simulink model "PV_MEV"  (R2025a)
settings: Solver=VariableStepAuto  StartTime=0.0  StopTime=1  RelTol=1e-3
InitFcn:
  | init_paras
model workspace (MAT data in the model file):
  atk_params = [0 1 0.85 999 0 50 0 0]
  atk_params_vdc = [0 1 0.85 999 0 50 0 0]
values from neighbouring files (symbols this model uses):
  C_PFC = 2600e-6    (= 0.0026)    [init_paras.m]
  ENABLE_HIL = 0    [init_paras.m]
  estimation_src = 1    [init_paras.m]
  Fnom = 50    [init_paras.m]
  Fr_I = Fnom*2    (= 100)    [init_paras.m]
  Ki_V = 80    [init_paras.m]
  Kp_I = 0.06    [init_paras.m]
  Kp_V = 0.25    [init_paras.m]
  Kr_I = 2.5    [init_paras.m]
  L_PFC = 600e-6    (= 0.0006)    [init_paras.m]
  Limit_V = 100    [init_paras.m]
  mm_10cycle_points = mm_points_per_cycle * 10    (= 800)    [init_paras.m]
  mm_fund_freq = 50    [init_paras.m]
  mm_points_per_cycle = 80    [init_paras.m]
  RL_PFC = 20e-3    (= 0.02)    [init_paras.m]
  Ro = 22.22    [init_paras.m]
  Ts_Control = 1/Fc    (= 5e-05)    [init_paras.m]
  Ts_Power = 50e-9    (= 5e-08)    [init_paras.m]
  use_d_predict = 1    [init_paras.m]
  use_harmonic = 1    [init_paras.m]
  use_p_predict = 0    [init_paras.m]
  Vnom_ac = 240    [init_paras.m]
undefined symbols (not defined in the file or in its folder): D1, Delta, DiscIntNeverNeededParam
libraries: spsSeriesRLCBranchLib x17, spsMeanLib x16, spsCurrentMeasurementLib x9, spsFourierLib x8, spsTHDLib x8, spsVoltageMeasurementLib x8, spsDiodeLib x7, MyLibrary x6, instrumentlib x6, pycoexlib x6, simulink x6, spsPWMGeneratorDCDCLib x4
(part 4 of 6)

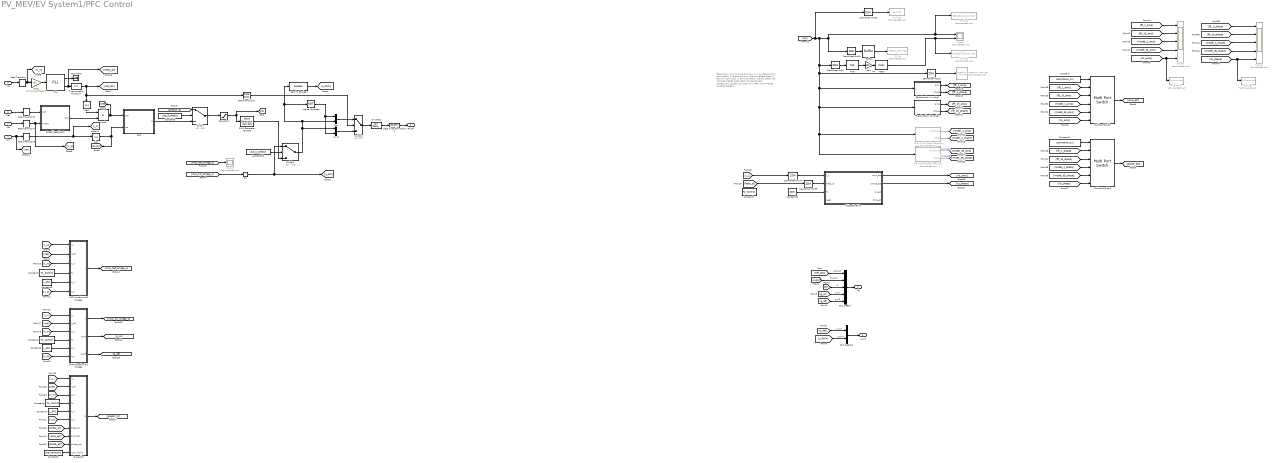
== system PV_MEV/EV System1/PFC Control ==
  note: Make sure
      | 1. onnxruntime and onnx in your base python enviroment.
      | 2. reload the onnx file and refresh them in the onnx call block.
      | or comment them like this
      | otherwise will lead matlab crash
      |
      | (bash)
      | conda activate matlab_onnx_py310
      | pip install onnx==1.14.0
      |
      | (matlab console)
      | target = "/home/changhong/anaconda3/envs/matlab_onnx_py310/bin/python";
      | pe = pyenv
      | pyenv("Version", target)
  Vref : Inport
  Vdc : Inport  Port=2
  Vac : Inport  Port=3
  Iac : Inport  Port=4
  AbsI : Abs  SaturateOnIntegerOverflow=off
  AbsV : Abs  SaturateOnIntegerOverflow=off
  Buffer : Buffer  N=80  V=79  OutputFrames=off
  Bus Creator : BusCreator  Inputs=5
  Bus Creator1 : BusCreator  Inputs=2
  Cast To Boolean : DataTypeConversion  OutDataTypeStr=boolean  SaturateOnIntegerOverflow=off  RndMeth=Floor
  Constant : Constant  Value=estimation_src
  Constant{1..2,4,6} (4 alike) : Constant  Value=Ts_Control
  Constant10 : Constant  Value=use_p_predict
  Constant11 : Constant  Value=estimation_src
  Constant12 : Constant  Value=4000
  Constant3 : Constant  Value=L_PFC
  Constant5 : Constant  Value=L_PFC
  Constant7 : Constant  Value=L_PFC
  Constant8 : Constant  Value=use_harmonic
  Constant9 : Constant  Value=use_d_predict
  D_predict : MATLAB Function  TreatAsAtomicUnit=on
  Data Type Conversion2 : DataTypeConversion  OutDataTypeStr=double  SaturateOnIntegerOverflow=off  RndMeth=Floor
  Gain : Gain  Gain=100
  Half Cycle Model Prediction : Subsystem  Commented=on
  Logical Operator : Logic  Operator=NOT  AllPortsSameDT=off  OutDataTypeStr=float('double')
  MCP Function Half bridge1 : MATLAB Function  TreatAsAtomicUnit=on
  Mean : spsMeanLib/Mean  Freq=50  Vinit=0  Ts=1/4000
  Multiport Switch : MultiPortSwitch  Inputs=5  SaturateOnIntegerOverflow=off  InputSameDT=off
  Multiport Switch1 : MultiPortSwitch  Inputs=5  SaturateOnIntegerOverflow=off  InputSameDT=off
  Mux : Mux  Inputs=2
  Mux2 : Mux  Inputs=2
  On Delay : spsOnDelayLib/On Delay  DelayType=On delay  delay=DT_PFC  ic=0  Ts=Ts_Power
  One  Cycle Model Prediction : Subsystem  Commented=on
  PLL : spsPLLLib/PLL  Fmin=0.9*Fnom  Par_Init=[0, Fnom]  ParK=[180, 3200, 1]  TcD=1e-4  MaxRateChangeFreq=12  FilterCutOffFreq=25  Ts=Ts_Control  AGC=on
  PR2 : Subsystem  mask(Current Regulator (Pr)){Kp=Kp_I, Kr=Kr_I, Fr=Fr_I}
      mask prompts: Kp "Proportional gain"; Kr "Resonant gain"; Fr "Resonant frequency (Hz)"
      mask help: This block implements a currentregulator using a PR controller.
      mask Display: disp('Current Regulator\n PR');
  PWM Generator (DC-DC) : spsPWMGeneratorDCDCLib/PWM Generator (DC-DC)  Fsw=Fsw  Ts=Ts_Power
  Prod1 : Product
  RLS_estimation : MATLAB Function  TreatAsAtomicUnit=on
  RT : RateTransition  OutPortSampleTime=5e-08
  Rate Transition{,3..5} (4 alike) : RateTransition  OutPortSampleTime=Ts_Control
  Rate Transition2 : RateTransition  OutPortSampleTime=Ts_Power
  Saturation : Saturate  UpperLimit=1  LowerLimit=0
  Scope : Scope  Commented=on  NumInputPorts=2
      settings: ActiveDisplayYMinimum=-211.219  ActiveDisplayYMaximum=223.7073  DataLoggingVariableName=ScopeData4  DataLoggingSaveFormat=Array
  Scope1 : Scope  Commented=on  NumInputPorts=5
      settings: ActiveDisplayYMinimum=-19.4864  ActiveDisplayYMaximum=175.3777  DataLoggingVariableName=ScopeData5  DataLoggingSaveFormat=Array
  Scope2 : Scope  Commented=on
      settings: DataLoggingVariableName=ScopeData9  DataLoggingSaveFormat=Array
  Scope3 : Scope  Commented=on  NumInputPorts=5
      settings: ActiveDisplayYMinimum=-3.927  ActiveDisplayYMaximum=3.927  DataLoggingVariableName=ScopeData6  DataLoggingSaveFormat=Array
  Spectrum Analyzer : SpectrumAnalyzer  Commented=on  WindowPosition=[-2559.000000,62.000000,1707.000000,996.000000,]  ScopeFrameLocation=window  SampleRateSource=Property  SampleRate=8000  PlotAsTwoSidedSpectrum=off  WindowInvariantSamplesPerUpdate=on  FrequencySpan=Start and stop frequencies  StartFrequency=0  StopFrequency=2000  YLimits=[-21.57310057,75.63654601]  ColorLimits=[-42.4528 59.157]
  Speed Regulator2 : Subsystem  DialogController=POWERSYS.PowerSysDialog  mask(Voltage Regulator){Kp=Kp_V, Ki=Ki_V, Limit_wreg=Limit_V, Init=0, Ts=Ts_Control}
      mask prompts: Kp "Proportional gain (Kp):"; Ki "Integral gain (Ki):"; Limit_wreg "Output limits"; Init "Output initial value:"; Ts "Sample time:"
      mask help: This block implements a voltage regulator using an ant-windup PI controller.
      mask Display: disp('Voltage\nRegulator');
  Switch : Switch  Criteria=u2 > Threshold  Threshold=0.5  SaturateOnIntegerOverflow=off  InputSameDT=off
  Switch1 : Switch  SaturateOnIntegerOverflow=off  InputSameDT=off
  Switch2 : Switch  Criteria=u2 > Threshold  Threshold=0.5  SaturateOnIntegerOverflow=off  InputSameDT=off
  THD : spsTHDLib/THD  Freq=50  Ts=1/4000
  Terminator : Terminator
  To File : ToFile  Commented=on  Filename=MPCC_IAC.mat  SaveFormat=Timeseries
  To File1 : ToFile  Commented=on  Filename=rls_phase.mat  SaveFormat=Timeseries
  To File2 : ToFile  Commented=on  Filename=rls_amp.mat  SaveFormat=Timeseries
  To File3 : ToFile  Commented=on  Filename=Iac.mat  SaveFormat=Timeseries
  To File4 : ToFile  Commented=on  Filename=results/Iac_ori.mat  SaveFormat=Timeseries
  To File5 : ToFile  Commented=on  Filename=results/THD_ori.mat  SaveFormat=Timeseries
  Trigonometric Function7 : Trigonometry
  UMPC Function Full bridge1 : MATLAB Function  TreatAsAtomicUnit=on
  Zero-Order Hold{,1,3..5} (5 alike) : ZeroOrderHold  SampleTime=1/4000
  Zero-Order Hold2 : ZeroOrderHold  SampleTime=1/8000
  fft estimation 1 cycle2 : Subsystem
  fft estimation 10 cycle2 : Subsystem
  to-pu : Gain  Gain=1/(Vnom_ac*sqrt(2))
  g1_g2 : Outport  PortDimensions=2
  Sig : Outport  Port=2
  u_swt : Outport  Port=3
  wires:
  Zero-Order Hold5/1 -> RLS_estimation/2(theta_pll)
  Zero-Order Hold4/1 -> RLS_estimation/1(i_L)
  Constant12/1 -> RLS_estimation/3(Ts)
  [i_L] -> Zero-Order Hold4/1
  Zero-Order Hold3/1 -> To File3/1
  [rls_phase] -> Scope3/5, To File1/1
  [model_05_phase] -> Scope3/4
  [model_1_phase] -> Scope3/3
  [fft_10_phase] -> Scope3/2
  [fft_1_phase] -> Scope3/1
  [rls_amp] -> Scope1/5, To File2/1
  [model_05_amp] -> Scope1/4
  [model_1_amp] -> Scope1/3
  [fft_10_amp] -> Scope1/2
  [fft_1_amp] -> Scope1/1
  Constant11/1 -> Multiport Switch1/1
  Multiport Switch1/1 -> [phase_est]
  [fft_1_phase] -> Multiport Switch1/2
  [fft_10_phase] -> Multiport Switch1/3
  [model_1_phase] -> Multiport Switch1/4
  [model_05_phase] -> Multiport Switch1/5
  [rls_phase] -> Multiport Switch1/6
  [rls_amp] -> Multiport Switch/6
  [model_05_amp] -> Multiport Switch/5
  [model_1_amp] -> Multiport Switch/4
  [fft_10_amp] -> Multiport Switch/3
  [fft_1_amp] -> Multiport Switch/2
  RLS_estimation/2(phase_est) -> [rls_phase]
  RLS_estimation/1(amp_est) -> [rls_amp]
  Multiport Switch/1 -> [amp_est]
  Half Cycle Model Prediction/2(phase) -> [model_05_phase]  "hase_est"
  Half Cycle Model Prediction/1(amplitude) -> [model_05_amp]  "amp_est"
  One  Cycle Model Prediction/2(phase) -> [model_1_phase]
  One  Cycle Model Prediction/1(amplitude) -> [model_1_amp]
  fft estimation 10 cycle2/2(phase) -> [fft_10_phase]
  fft estimation 10 cycle2/1(amp) -> [fft_10_amp]
  fft estimation 1 cycle2/2(phase) -> [fft_1_phase]
  fft estimation 1 cycle2/1(amp) -> [fft_1_amp]
  Constant/1 -> Multiport Switch/1
  Logical Operator/1 -> Mux/1, Mux2/2
  Constant10/1 -> Switch2/2
  Switch/1 -> Saturation/1
  PR2/1(D) -> Switch/3
  [predict_D] -> Switch/1
  Constant9/1 -> Switch/2
  [mcp_half_bridge_o] -> Scope2/1
  D_predict/1(D) -> [predict_D]
  [theta_pll] -> D_predict/7(theta_pll)
  Constant8/1 -> D_predict/10(use_harmonic)
  [phase_est] -> D_predict/9(phase_est)
  [amp_est] -> D_predict/8(amp_est)
  [V_o] -> D_predict/6(V_o)
  Constant7/1 -> D_predict/5(L_in)
  Constant6/1 -> D_predict/4(Ts)
  [V_in] -> D_predict/3(V_in)
  [Iref] -> D_predict/2(i_ref)
  [i_L] -> D_predict/1(i_L)
  [theta_pll] -> Zero-Order Hold5/1
  [g_off] -> Bus Creator/5  "g_off"
  [g_on] -> Bus Creator/4  "g_on"
  UMPC Function Full bridge1/3(g_off) -> [g_off]
  UMPC Function Full bridge1/2(g_on) -> [g_on]
  UMPC Function Full bridge1/1(y) -> [mcp_full_bridge_o]
  [V_o] -> UMPC Function Full bridge1/6(V_o)
  Constant5/1 -> UMPC Function Full bridge1/5(L_in)
  Constant4/1 -> UMPC Function Full bridge1/4(Ts)
  [V_in] -> UMPC Function Full bridge1/3(V_in)
  [Iref] -> UMPC Function Full bridge1/2(i_ref)
  [i_L] -> UMPC Function Full bridge1/1(i_L)
  MCP Function Half bridge1/1(y) -> [mcp_half_bridge_o]
  [V_o] -> MCP Function Half bridge1/6(V_o)
  Constant3/1 -> MCP Function Half bridge1/5(L_in)
  Constant2/1 -> MCP Function Half bridge1/4(Ts)
  [V_in] -> MCP Function Half bridge1/3(V_in)
  [Iref] -> MCP Function Half bridge1/2(i_ref)
  [i_L] -> MCP Function Half bridge1/1(i_L)
  Zero-Order Hold1/1 -> Buffer/1
  THD/1 -> Gain/1
  Zero-Order Hold2/1 -> Spectrum Analyzer/1
  Mean/1 -> Scope/2, To File5/1
  Zero-Order Hold/1 -> THD/1
  Gain/1 -> Mean/1
  Buffer/1 -> To File/1
  [Iac] -> Scope/1, To File4/1, Zero-Order Hold1/1, Zero-Order Hold/1, Zero-Order Hold2/1, fft estimation 1 cycle2/1(u), fft estimation 10 cycle2/1(u), One  Cycle Model Prediction/1(u), Half Cycle Model Prediction/1(u), Zero-Order Hold3/1  "Iac"
  [u_PWM] -> Bus Creator1/2  "u_PWM"
  On Delay/1 -> Data Type Conversion2/1
  Vref/1 -> Rate Transition3/1
  Switch2/1 -> Mux2/1, Mux/2, Cast To Boolean/1, Logical Operator/1
  [Iac_abs] -> Bus Creator/2  "Iac_abc"
  AbsV/1 -> Prod1/1
  PLL/1 -> Terminator/1
  Rate Transition5/1 -> AbsI/1, [i_L]
  Bus Creator/1 -> Sig/1
  Prod1/1 -> PR2/1(Iref), [Iref]
  Vac/1 -> Rate Transition/1
  PWM Generator (DC-DC)/1 -> Switch2/3
  Cast To Boolean/1 -> [u_PWM]
  RT/1 -> [u_obs], Switch2/1
  [Iref_obs] -> Bus Creator/1  "Iref_obs"
  [mcp_full_bridge_o] -> RT/1
  Vdc/1 -> Rate Transition4/1
  Mux2/1 -> Switch1/3
  [u_obs] -> Bus Creator1/1  "u_obs"
  Rate Transition4/1 -> [V_o], Speed Regulator2/2(Vmeas)
  Switch1/1 -> On Delay/1
  Rate Transition3/1 -> Speed Regulator2/1(Vref)
  [D] -> Bus Creator/3  "D"
  Trigonometric Function7/1 -> [Iref_obs], Rate Transition2/1, AbsV/1
  AbsI/1 -> [Iac_abs], PR2/2(Iac)
  Bus Creator1/1 -> u_swt/1
  Rate Transition/1 -> to-pu/1, [V_in]
  to-pu/1 -> PLL/1
  Saturation/1 -> [D], PWM Generator (DC-DC)/1
  PLL/2 -> Trigonometric Function7/1, [theta_pll]
  Data Type Conversion2/1 -> g1_g2/1
  Rate Transition2/1 -> Switch1/2
  Speed Regulator2/1(Out) -> Prod1/2
  Iac/1 -> Rate Transition5/1, [Iac]
  Mux/1 -> Switch1/1

== system PV_MEV/EV System1/Subsystem ==

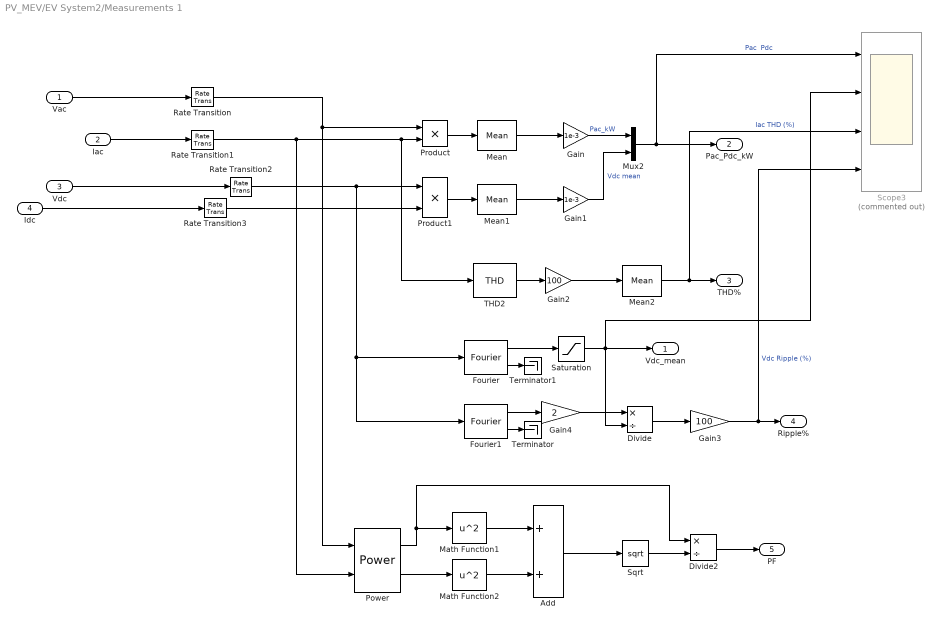
== system PV_MEV/EV System2/Measurements 1 ==
  Vac : Inport
  Iac : Inport  Port=2
  Vdc : Inport  Port=3
  Idc : Inport  Port=4
  Add : Sum
  Divide : Product  Inputs=*/
  Divide2 : Product  Inputs=*/
  Fourier : spsFourierLib/Fourier  Freq=Fnom  n=0  InInit=[0, 0]  Ts=Ts_Control
  Fourier1 : spsFourierLib/Fourier  Freq=Fnom  n=2  InInit=[0, 0]  Ts=Ts_Control
  Gain : Gain  Gain=1e-3
  Gain1 : Gain  Gain=1e-3
  Gain2 : Gain  Gain=100
  Gain3 : Gain  Gain=100
  Gain4 : Gain  Gain=2
  Math Function1 : Math  Operator=square
  Math Function2 : Math  Operator=square
  Mean : spsMeanLib/Mean  Freq=Fnom  Vinit=0  Ts=Ts_Control
  Mean1 : spsMeanLib/Mean  Freq=Fnom  Vinit=0  Ts=Ts_Control
  Mean2 : spsMeanLib/Mean  Freq=Fnom  Vinit=0  Ts=Ts_Control
  Mux2 : Mux  Inputs=2
  Power : spsPowerLib/Power  Freq=Fnom  Vinit=[1, 0]  Iinit=[1, 0]  Ts=Ts_Control
  Product : Product
  Product1 : Product
  Rate Transition{,1..3} (4 alike) : RateTransition  OutPortSampleTime=Ts_Control
  Saturation : Saturate  UpperLimit=inf  LowerLimit=eps
  Scope3 : Scope  Commented=on  NumInputPorts=4
      settings: DataLoggingSaveFormat=Array
  Sqrt : Sqrt
  THD2 : spsTHDLib/THD  Freq=Fnom  Ts=Ts_Control
  Terminator : Terminator
  Terminator1 : Terminator
  Vdc_mean : Outport
  Pac_Pdc_kW : Outport  Port=2
  THD% : Outport  Port=3
  Ripple% : Outport  Port=4
  PF : Outport  Port=5
  wires:
  Gain1/1 -> Mux2/2  "Vdc mean"
  Product1/1 -> Mean1/1
  Mean/1 -> Gain/1
  Product/1 -> Mean/1
  Gain/1 -> Mux2/1  "Pac_kW"
  THD2/1 -> Gain2/1
  Mean1/1 -> Gain1/1
  Iac/1 -> Rate Transition1/1
  Mux2/1 -> Scope3/1, Pac_Pdc_kW/1  "Pac  Pdc"
  Gain2/1 -> Mean2/1
  Mean2/1 -> Scope3/3, THD%/1  "Iac THD (%)"
  Fourier/2 -> Terminator1/1
  Fourier/1 -> Saturation/1
  Saturation/1 -> Scope3/2, Vdc_mean/1, Divide/2
  Divide/1 -> Gain3/1
  Fourier1/1 -> Gain4/1
  Gain4/1 -> Divide/1
  Fourier1/2 -> Terminator/1
  Gain3/1 -> Scope3/4, Ripple%/1  "Vdc Ripple (%)"
  Power/1 -> Math Function1/1, Divide2/1
  Power/2 -> Math Function2/1
  Math Function1/1 -> Add/1
  Math Function2/1 -> Add/2
  Add/1 -> Sqrt/1
  Sqrt/1 -> Divide2/2
  Divide2/1 -> PF/1
  Rate Transition1/1 -> Power/2, THD2/1, Product/2
  Vdc/1 -> Rate Transition2/1
  Idc/1 -> Rate Transition3/1
  Rate Transition/1 -> Power/1, Product/1
  Vac/1 -> Rate Transition/1
  Rate Transition2/1 -> Product1/1, Fourier/1, Fourier1/1
  Rate Transition3/1 -> Product1/2

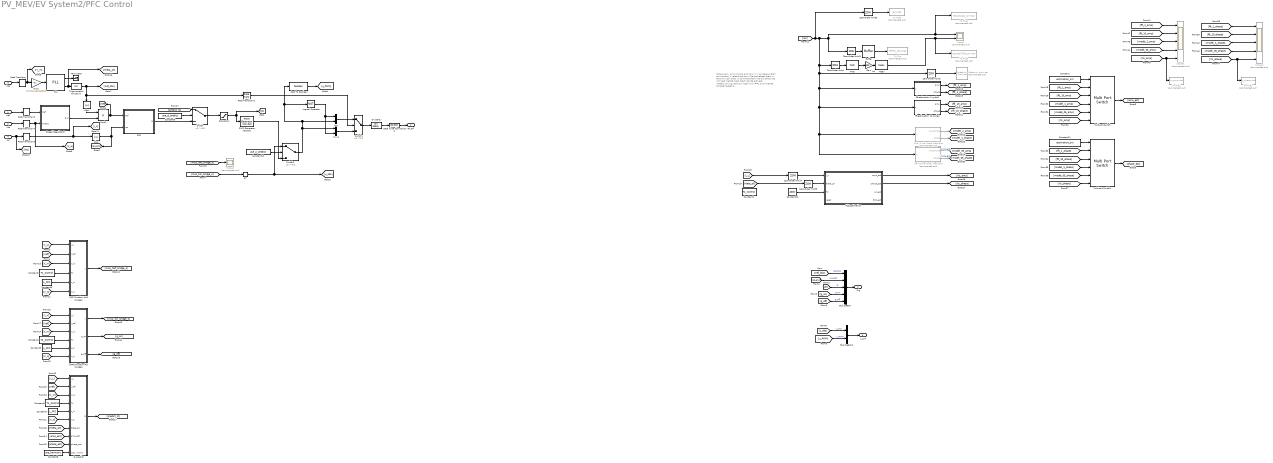
== system PV_MEV/EV System2/PFC Control ==
  note: Make sure
      | 1. onnxruntime and onnx in your base python enviroment.
      | 2. reload the onnx file and refresh them in the onnx call block.
      | or comment them like this
      | otherwise will lead matlab crash
      |
      | (bash)
      | conda activate matlab_onnx_py310
      | pip install onnx==1.14.0
      |
      | (matlab console)
      | target = "/home/changhong/anaconda3/envs/matlab_onnx_py310/bin/python";
      | pe = pyenv
      | pyenv("Version", target)
  Vref : Inport
  Vdc : Inport  Port=2
  Vac : Inport  Port=3
  Iac : Inport  Port=4
  AbsI : Abs  SaturateOnIntegerOverflow=off
  AbsV : Abs  SaturateOnIntegerOverflow=off
  Buffer : Buffer  N=80  V=79  OutputFrames=off
  Bus Creator : BusCreator  Inputs=5
  Bus Creator1 : BusCreator  Inputs=2
  Cast To Boolean : DataTypeConversion  OutDataTypeStr=boolean  SaturateOnIntegerOverflow=off  RndMeth=Floor
  Constant : Constant  Value=estimation_src
  Constant{1..2,4,6} (4 alike) : Constant  Value=Ts_Control
  Constant10 : Constant  Value=use_p_predict
  Constant11 : Constant  Value=estimation_src
  Constant12 : Constant  Value=4000
  Constant3 : Constant  Value=L_PFC
  Constant5 : Constant  Value=L_PFC
  Constant7 : Constant  Value=L_PFC
  Constant8 : Constant  Value=use_harmonic
  Constant9 : Constant  Value=use_d_predict
  D_predict : MATLAB Function  TreatAsAtomicUnit=on
  Data Type Conversion2 : DataTypeConversion  OutDataTypeStr=double  SaturateOnIntegerOverflow=off  RndMeth=Floor
  Gain : Gain  Gain=100
  Half Cycle Model Prediction : Subsystem  Commented=on
  Logical Operator : Logic  Operator=NOT  AllPortsSameDT=off  OutDataTypeStr=float('double')
  MCP Function Half bridge1 : MATLAB Function  TreatAsAtomicUnit=on
  Mean : spsMeanLib/Mean  Freq=50  Vinit=0  Ts=1/4000
  Multiport Switch : MultiPortSwitch  Inputs=5  SaturateOnIntegerOverflow=off  InputSameDT=off
  Multiport Switch1 : MultiPortSwitch  Inputs=5  SaturateOnIntegerOverflow=off  InputSameDT=off
  Mux : Mux  Inputs=2
  Mux2 : Mux  Inputs=2
  On Delay : spsOnDelayLib/On Delay  DelayType=On delay  delay=DT_PFC  ic=0  Ts=Ts_Power
  One  Cycle Model Prediction : Subsystem  Commented=on
  PLL : spsPLLLib/PLL  Fmin=0.9*Fnom  Par_Init=[0, Fnom]  ParK=[180, 3200, 1]  TcD=1e-4  MaxRateChangeFreq=12  FilterCutOffFreq=25  Ts=Ts_Control  AGC=on
  PR2 : Subsystem  mask(Current Regulator (Pr)){Kp=Kp_I, Kr=Kr_I, Fr=Fr_I}
      mask prompts: Kp "Proportional gain"; Kr "Resonant gain"; Fr "Resonant frequency (Hz)"
      mask help: This block implements a currentregulator using a PR controller.
      mask Display: disp('Current Regulator\n PR');
  PWM Generator (DC-DC) : spsPWMGeneratorDCDCLib/PWM Generator (DC-DC)  Fsw=Fsw  Ts=Ts_Power
  Prod1 : Product
  RLS_estimation : MATLAB Function  TreatAsAtomicUnit=on
  RT : RateTransition  OutPortSampleTime=5e-08
  Rate Transition{,3..5} (4 alike) : RateTransition  OutPortSampleTime=Ts_Control
  Rate Transition2 : RateTransition  OutPortSampleTime=Ts_Power
  Saturation : Saturate  UpperLimit=1  LowerLimit=0
  Scope : Scope  Commented=on  NumInputPorts=2
      settings: ActiveDisplayYMinimum=-211.219  ActiveDisplayYMaximum=223.7073  DataLoggingVariableName=ScopeData4  DataLoggingSaveFormat=Array
  Scope1 : Scope  Commented=on  NumInputPorts=5
      settings: ActiveDisplayYMinimum=-19.4864  ActiveDisplayYMaximum=175.3777  DataLoggingVariableName=ScopeData5  DataLoggingSaveFormat=Array
  Scope2 : Scope  Commented=on
      settings: DataLoggingVariableName=ScopeData9  DataLoggingSaveFormat=Array
  Scope3 : Scope  Commented=on  NumInputPorts=5
      settings: ActiveDisplayYMinimum=-3.927  ActiveDisplayYMaximum=3.927  DataLoggingVariableName=ScopeData6  DataLoggingSaveFormat=Array
  Spectrum Analyzer : SpectrumAnalyzer  Commented=on  WindowPosition=[-2559.000000,62.000000,1707.000000,996.000000,]  ScopeFrameLocation=window  SampleRateSource=Property  SampleRate=8000  PlotAsTwoSidedSpectrum=off  WindowInvariantSamplesPerUpdate=on  FrequencySpan=Start and stop frequencies  StartFrequency=0  StopFrequency=2000  YLimits=[-21.57310057,75.63654601]  ColorLimits=[-42.4528 59.157]
  Speed Regulator2 : Subsystem  DialogController=POWERSYS.PowerSysDialog  mask(Voltage Regulator){Kp=Kp_V, Ki=Ki_V, Limit_wreg=Limit_V, Init=0, Ts=Ts_Control}
      mask prompts: Kp "Proportional gain (Kp):"; Ki "Integral gain (Ki):"; Limit_wreg "Output limits"; Init "Output initial value:"; Ts "Sample time:"
      mask help: This block implements a voltage regulator using an ant-windup PI controller.
      mask Display: disp('Voltage\nRegulator');
  Switch : Switch  Criteria=u2 > Threshold  Threshold=0.5  SaturateOnIntegerOverflow=off  InputSameDT=off
  Switch1 : Switch  SaturateOnIntegerOverflow=off  InputSameDT=off
  Switch2 : Switch  Criteria=u2 > Threshold  Threshold=0.5  SaturateOnIntegerOverflow=off  InputSameDT=off
  THD : spsTHDLib/THD  Freq=50  Ts=1/4000
  Terminator : Terminator
  To File : ToFile  Commented=on  Filename=MPCC_IAC.mat  SaveFormat=Timeseries
  To File1 : ToFile  Commented=on  Filename=rls_phase.mat  SaveFormat=Timeseries
  To File2 : ToFile  Commented=on  Filename=rls_amp.mat  SaveFormat=Timeseries
  To File3 : ToFile  Commented=on  Filename=Iac.mat  SaveFormat=Timeseries
  To File4 : ToFile  Commented=on  Filename=results/Iac_ori.mat  SaveFormat=Timeseries
  To File5 : ToFile  Commented=on  Filename=results/THD_ori.mat  SaveFormat=Timeseries
  Trigonometric Function7 : Trigonometry
  UMPC Function Full bridge1 : MATLAB Function  TreatAsAtomicUnit=on
  Zero-Order Hold{,1,3..5} (5 alike) : ZeroOrderHold  SampleTime=1/4000
  Zero-Order Hold2 : ZeroOrderHold  SampleTime=1/8000
  fft estimation 1 cycle2 : Subsystem
  fft estimation 10 cycle2 : Subsystem
  to-pu : Gain  Gain=1/(Vnom_ac*sqrt(2))
  g1_g2 : Outport  PortDimensions=2
  Sig : Outport  Port=2
  u_swt : Outport  Port=3
  wires:
  Mux/1 -> Switch1/1
  Iac/1 -> [Iac], Rate Transition5/1
  Speed Regulator2/1(Out) -> Prod1/2
  Rate Transition2/1 -> Switch1/2
  Data Type Conversion2/1 -> g1_g2/1
  PLL/2 -> [theta_pll], Trigonometric Function7/1
  Saturation/1 -> PWM Generator (DC-DC)/1, [D]
  to-pu/1 -> PLL/1
  Rate Transition/1 -> [V_in], to-pu/1
  Bus Creator1/1 -> u_swt/1
  AbsI/1 -> PR2/2(Iac), [Iac_abs]
  Trigonometric Function7/1 -> AbsV/1, Rate Transition2/1, [Iref_obs]
  [D] -> Bus Creator/3  "D"
  Rate Transition3/1 -> Speed Regulator2/1(Vref)
  Switch1/1 -> On Delay/1
  Rate Transition4/1 -> Speed Regulator2/2(Vmeas), [V_o]
  [u_obs] -> Bus Creator1/1  "u_obs"
  Mux2/1 -> Switch1/3
  Vdc/1 -> Rate Transition4/1
  [mcp_full_bridge_o] -> RT/1
  [Iref_obs] -> Bus Creator/1  "Iref_obs"
  RT/1 -> Switch2/1, [u_obs]
  Cast To Boolean/1 -> [u_PWM]
  PWM Generator (DC-DC)/1 -> Switch2/3
  Vac/1 -> Rate Transition/1
  Prod1/1 -> [Iref], PR2/1(Iref)
  Bus Creator/1 -> Sig/1
  Rate Transition5/1 -> [i_L], AbsI/1
  PLL/1 -> Terminator/1
  AbsV/1 -> Prod1/1
  [Iac_abs] -> Bus Creator/2  "Iac_abc"
  Switch2/1 -> Logical Operator/1, Cast To Boolean/1, Mux/2, Mux2/1
  Vref/1 -> Rate Transition3/1
  On Delay/1 -> Data Type Conversion2/1
  [u_PWM] -> Bus Creator1/2  "u_PWM"
  [Iac] -> Zero-Order Hold3/1, Half Cycle Model Prediction/1(u), One  Cycle Model Prediction/1(u), fft estimation 10 cycle2/1(u), fft estimation 1 cycle2/1(u), Zero-Order Hold2/1, Zero-Order Hold/1, Zero-Order Hold1/1, To File4/1, Scope/1  "Iac"
  Buffer/1 -> To File/1
  Gain/1 -> Mean/1
  Zero-Order Hold/1 -> THD/1
  Mean/1 -> To File5/1, Scope/2
  Zero-Order Hold2/1 -> Spectrum Analyzer/1
  THD/1 -> Gain/1
  Zero-Order Hold1/1 -> Buffer/1
  [i_L] -> MCP Function Half bridge1/1(i_L)
  [Iref] -> MCP Function Half bridge1/2(i_ref)
  [V_in] -> MCP Function Half bridge1/3(V_in)
  Constant2/1 -> MCP Function Half bridge1/4(Ts)
  Constant3/1 -> MCP Function Half bridge1/5(L_in)
  [V_o] -> MCP Function Half bridge1/6(V_o)
  MCP Function Half bridge1/1(y) -> [mcp_half_bridge_o]
  [i_L] -> UMPC Function Full bridge1/1(i_L)
  [Iref] -> UMPC Function Full bridge1/2(i_ref)
  [V_in] -> UMPC Function Full bridge1/3(V_in)
  Constant4/1 -> UMPC Function Full bridge1/4(Ts)
  Constant5/1 -> UMPC Function Full bridge1/5(L_in)
  [V_o] -> UMPC Function Full bridge1/6(V_o)
  UMPC Function Full bridge1/1(y) -> [mcp_full_bridge_o]
  UMPC Function Full bridge1/2(g_on) -> [g_on]
  UMPC Function Full bridge1/3(g_off) -> [g_off]
  [g_on] -> Bus Creator/4  "g_on"
  [g_off] -> Bus Creator/5  "g_off"
  [theta_pll] -> Zero-Order Hold5/1
  [i_L] -> D_predict/1(i_L)
  [Iref] -> D_predict/2(i_ref)
  [V_in] -> D_predict/3(V_in)
  Constant6/1 -> D_predict/4(Ts)
  Constant7/1 -> D_predict/5(L_in)
  [V_o] -> D_predict/6(V_o)
  [amp_est] -> D_predict/8(amp_est)
  [phase_est] -> D_predict/9(phase_est)
  Constant8/1 -> D_predict/10(use_harmonic)
  [theta_pll] -> D_predict/7(theta_pll)
  D_predict/1(D) -> [predict_D]
  [mcp_half_bridge_o] -> Scope2/1
  Constant9/1 -> Switch/2
  [predict_D] -> Switch/1
  PR2/1(D) -> Switch/3
  Switch/1 -> Saturation/1
  Constant10/1 -> Switch2/2
  Logical Operator/1 -> Mux2/2, Mux/1
  Constant/1 -> Multiport Switch/1
  fft estimation 1 cycle2/1(amp) -> [fft_1_amp]
  fft estimation 1 cycle2/2(phase) -> [fft_1_phase]
  fft estimation 10 cycle2/1(amp) -> [fft_10_amp]
  fft estimation 10 cycle2/2(phase) -> [fft_10_phase]
  One  Cycle Model Prediction/1(amplitude) -> [model_1_amp]
  One  Cycle Model Prediction/2(phase) -> [model_1_phase]
  Half Cycle Model Prediction/1(amplitude) -> [model_05_amp]  "amp_est"
  Half Cycle Model Prediction/2(phase) -> [model_05_phase]  "hase_est"
  Multiport Switch/1 -> [amp_est]
  RLS_estimation/1(amp_est) -> [rls_amp]
  RLS_estimation/2(phase_est) -> [rls_phase]
  [fft_1_amp] -> Multiport Switch/2
  [fft_10_amp] -> Multiport Switch/3
  [model_1_amp] -> Multiport Switch/4
  [model_05_amp] -> Multiport Switch/5
  [rls_amp] -> Multiport Switch/6
  [rls_phase] -> Multiport Switch1/6
  [model_05_phase] -> Multiport Switch1/5
  [model_1_phase] -> Multiport Switch1/4
  [fft_10_phase] -> Multiport Switch1/3
  [fft_1_phase] -> Multiport Switch1/2
  Multiport Switch1/1 -> [phase_est]
  Constant11/1 -> Multiport Switch1/1
  [fft_1_amp] -> Scope1/1
  [fft_10_amp] -> Scope1/2
  [model_1_amp] -> Scope1/3
  [model_05_amp] -> Scope1/4
  [rls_amp] -> To File2/1, Scope1/5
  [fft_1_phase] -> Scope3/1
  [fft_10_phase] -> Scope3/2
  [model_1_phase] -> Scope3/3
  [model_05_phase] -> Scope3/4
  [rls_phase] -> To File1/1, Scope3/5
  Zero-Order Hold3/1 -> To File3/1
  [i_L] -> Zero-Order Hold4/1
  Constant12/1 -> RLS_estimation/3(Ts)
  Zero-Order Hold4/1 -> RLS_estimation/1(i_L)
  Zero-Order Hold5/1 -> RLS_estimation/2(theta_pll)

== system PV_MEV/EV System2/Subsystem ==

== system PV_MEV/PV System/DC AC Inverter ==
  note: 500V
      | 3-level VSC
  3-Level Bridge : spsThreeLevelBridgeLib/Three-Level Bridge  Arms=3  SnubberResistance=1e6  SbubberCapacitance=inf  Device=IGBT / Diodes  Ron=0.2e-3  ForwardVoltages="[  0  0 ]"  Measurements=None
      settings: AttributesFormatString=\n
  Deblock Converters : Step  Time=0.05  SampleTime=0
  Product1 : Product  RndMeth=Zero
  VSC Control : Subsystem  mask(VSC Main Controller){nom=[ 100e3  Fnom ], Vnom=[ 25e3 Vnom_ac ], Vnom_dc=500, RLxfo=[0.002  0.06 ], RLchoke=[2e-3  250e-6  ], K_VDCreg=[7  800], K_Ireg=[0.3 20], Ts=Ts_Control}
      mask prompts: nom "Nominal power and frequency [ Pnom(VA)  Fnom(Hz) ]:"; Vnom "Nominal primary and secondary voltages (Vrms LL) [ Vnom_prim   Vnom_sec ]:"; Vnom_dc "Nominal DC bus voltage (V):"; RLxfo "Total transformer leakage impedance (pu/Pnom) [ Rxfo  Lxf ]"; RLchoke "Choke impedance [ R(ohm) L(H) ]"; K_VDCreg "VDC regultator gains [ Kp  Ki ]:"; K_Ireg "Current regulator gains [ Kp  Ki ]:"; Ts "Sample time"
      mask init:
      | Pnom=nom(1);
      | Fnom=nom(2);
      | Vnom_prim=Vnom(1);
      | Vnom_sec=Vnom(2);
      | Zbase=Vnom_sec^2/Pnom;
      | Rtot_pu=RLxfo(1) + RLchoke(1)/Zbase;
      | Ltot_pu=RLxfo(2) + RLchoke(2)/(Zbase/(2*pi*Fnom));
      | Kp_VDCreg=K_VDCreg(1);
      | Ki_VDCreg=K_VDCreg(2);
      | Kp_Ireg=K_Ireg(1);
      | Ki_Ireg=K_Ireg(2);
      | Vdc_ref=Vnom_dc;
      | % Used to determine initial value of Boost Control (MPPT)
      | assignin('base','Vdc_ref_Inv',Vdc_ref);
  DC + IN : PMIOPort  Side=Left
  DC Mid IN : PMIOPort  Port=2  Side=Left
  DC - IN : PMIOPort  Port=3  Side=Left
  A : PMIOPort  Port=4  Side=Right
  B : PMIOPort  Port=5  Side=Right
  C : PMIOPort  Port=6  Side=Right
  wires:
  [Iabc_B1] -> VSC Control/2(Iabc_prim)
  VSC Control/1(Pulses) -> Product1/2
  [Vdc] -> VSC Control/3(Vdc_mes)
  [Vabc_B1] -> VSC Control/1(Vabc_prim)
  Product1/1 -> 3-Level Bridge/1
  Deblock Converters/1 -> Product1/1
  connections:
  DC + IN/RConn1 -- 3-Level Bridge/RConn1
  DC Mid IN/RConn1 -- 3-Level Bridge/RConn2
  DC - IN/RConn1 -- 3-Level Bridge/RConn3
  3-Level Bridge/LConn1 -- A/RConn1
  3-Level Bridge/LConn2 -- B/RConn1
  3-Level Bridge/LConn3 -- C/RConn1

== system PV_MEV/PV System/DC DC Boost Converter ==
  note: 5 kHz - 500V
      | Boost Converter
  C1 : spsSeriesRLCBranchLib/Series RLC Branch  LConnTagsString=__new0  RConnTagsString=__new0  BranchType=C  Resistance=1.0  Inductance=1.0  SetiL0=off  InitialCurrent=0  Capacitance=12000e-06  Setx0=off  InitialVoltage=0  Measurements=None
  C2 : spsSeriesRLCBranchLib/Series RLC Branch  LConnTagsString=__new0  RConnTagsString=__new0  BranchType=C  Resistance=1.0  Inductance=1.0  SetiL0=off  InitialCurrent=0  Capacitance=12000e-06  Setx0=off  InitialVoltage=0  Measurements=None
  C3 : spsSeriesRLCBranchLib/Series RLC Branch  LConnTagsString=__new0  RConnTagsString=__new0  BranchType=C  Resistance=1.0  Inductance=1.0  SetiL0=off  InitialCurrent=0  Capacitance=100e-6  Setx0=off  InitialVoltage=0  Measurements=Branch voltage
  Deblock Converters : Step  Time=0.05  SampleTime=0
  Diode1 : spsDiodeLib/Diode  Ron=1e-4  Lon=0  Vf=0  IC=0  UseSnubber=off  Rs=inf  Cs=inf  Measurements=off
  Display : Display
  IGBT1 : spsIGBTLib/IGBT  Ron=0.001  Lon=0  Vf=0  Tf=0  Tt=0  IC=0  Rs=1e5  Cs=inf  Measurements=off
  L1 : spsSeriesRLCBranchLib/Series RLC Branch  LConnTagsString=__new0  RConnTagsString=__new0  BranchType=RL  Resistance=0.005  Inductance=5e-3  SetiL0=off  InitialCurrent=0  Capacitance=1e-6  Setx0=off  InitialVoltage=0  Measurements=None
  "MPPT Controller using  'Incremental Conductance + Integral Regulator'  technique " : Subsystem  mask(Boost Control - MPPT){fc=5000, T_MPPT=200e-6, Dinit=0.5}
      mask prompts: fc "PWM switching frequency (Hz)"; T_MPPT "Time window used by MPPT control (s)"; Dinit "Initial value of duty cycle"
  Product2 : Product  RndMeth=Zero
  "Vdc " : spsVoltageMeasurementLib/Voltage Measurement  Tag=PoWeRsYsTeMmEaSuReMeNt  PhasorSimulation=off  OutputType=Magnitude  PSBequivalent=0
  PV DC IN + : PMIOPort  Side=Left
  PV DC IN - : PMIOPort  Port=2  Side=Left
  BC DC OUT + : PMIOPort  Port=3  Side=Right
  BC DC MID : PMIOPort  Port=4  Side=Right
  BC DC OUT - : PMIOPort  Port=5  Side=Right
  tag scope: Vdc=global
  wires:
  Product2/1 -> IGBT1/1
  "Vdc "/1 -> Display/1, [Vdc]
  "MPPT Controller using  'Incremental Conductance + Integral Regulator'  technique "/1(Pulses) -> Product2/2
  Deblock Converters/1 -> Product2/1
  [V_PV] -> "MPPT Controller using  'Incremental Conductance + Integral Regulator'  technique "/1(V_PV)
  [I_PV] -> "MPPT Controller using  'Incremental Conductance + Integral Regulator'  technique "/2(I_PV)
  connections:
  Diode1/RConn1 -- "Vdc "/LConn1 -- C1/LConn1 -- BC DC OUT +/RConn1
  PV DC IN -/RConn1 -- C3/RConn1 -- IGBT1/RConn1 -- "Vdc "/LConn2 -- C2/RConn1 -- BC DC OUT -/RConn1
  L1/RConn1 -- Diode1/LConn1 -- IGBT1/LConn1
  C2/LConn1 -- C1/RConn1 -- BC DC MID/RConn1
  PV DC IN +/RConn1 -- C3/LConn1 -- L1/LConn1

== system PV_MEV/PV System/PV Enviroment ==
  Irradiance (W/m^2) : Display
  Irradiance Temp : SignalEditorBlockLib/Signal Editor  FileName=PVArrayGridData.mat  ActiveScenario=Ramp_up_down_Irradiance  ActiveSignal=Temp  IsBus=off  OutputBusObjectStr=Bus: BusObject  SampleTime=0  OutputAfterFinalValue=Extrapolation  Unit=inherit  PreserveSignalName=on  ApplySigPropsToAllScenarios=on  ApplySigPropsToAllSignals=off  SignalPropertySource=Dialog parameters
  Temperature (deg. C) : Display
  Ir : Outport
  Temp : Outport  Port=2
  wires:
  Irradiance Temp/1 -> Irradiance (W/m^2)/1, Ir/1
  ? -> Temperature (deg. C)/1, Temp/1

== system PV_MEV/PV System/PV Status ==
  m_PV : Inport
  Bus Selector : BusSelector  OutputSignals=V_PV,I_PV,I_diode,Irradiance (W/m2),Temperature (deg C)
  tag scope: I_PV=global, Idiode_PV=global, Ir=global, Temp=global, V_PV=global
  wires:
  Bus Selector/5 -> [Temp]  "<Temperature (deg C)>"
  Bus Selector/3 -> [Idiode_PV]  "<I_diode>"
  Bus Selector/2 -> [I_PV]  "<I_PV>"
  m_PV/1 -> Bus Selector/1
  Bus Selector/4 -> [Ir]  "<Irradiance (W/m2)>"
  Bus Selector/1 -> [V_PV]  "<V_PV>"

== system PV_MEV/EV System/PFC Control/Enabled Subsystem ==
  Iac : Inport
  Data Type Conversion : DataTypeConversion  OutDataTypeStr=single  SaturateOnIntegerOverflow=off  RndMeth=Floor
  FFT Peak Hz : Display
  FFT Peak Receive : instrumentlib/TCP//IP Receive  Priority=20  Commented=on  Host=134.226.86.100  Port=5003  DataSize=[1, 1]  DataType=single  ASCIIFormatting=%f  Terminator=LF  CustomTerminator=10  ByteOrder=little-endian  EnableBlockingMode=on  Timeout=10  SampleTime=1/4000  SimulateUsing=Interpreted execution
  FFT TCP Send : instrumentlib/TCP//IP Send  Priority=-9  Commented=on  Host=134.226.86.100  Port=5002  ByteOrder=little-endian  EnableBlockingMode=on  Timeout=10  TransferDelay=off  SimulateUsing=Interpreted execution
  Scope1 : Scope  NumInputPorts=3
      settings: ActiveDisplayYMinimum=-294.38007890894539  ActiveDisplayYMaximum=319.34047090271997  DataLoggingVariableName=ScopeData8
  TCP Sample Hold : ZeroOrderHold  SampleTime=1/4000
  TCP/IP Receive1 : instrumentlib/TCP//IP Receive  Priority=10  Commented=on  Host=134.226.86.100  Port=5001  DataSize=[1, 1]  DataType=single  ASCIIFormatting=%f  Terminator=LF  CustomTerminator=10  ByteOrder=little-endian  EnableBlockingMode=on  Timeout=10  SampleTime=1/4000  SimulateUsing=Interpreted execution
  TCP/IP Send1 : instrumentlib/TCP//IP Send  Priority=-10  Commented=on  Host=134.226.86.100  Port=5000  ByteOrder=little-endian  EnableBlockingMode=on  Timeout=10  TransferDelay=off  SimulateUsing=Interpreted execution
  wires:
  Data Type Conversion/1 -> Scope1/2, TCP/IP Send1/1, FFT TCP Send/1
  Iac/1 -> Scope1/1, TCP Sample Hold/1
  TCP Sample Hold/1 -> Data Type Conversion/1
  FFT Peak Receive/1 -> FFT Peak Hz/1
  TCP/IP Receive1/1 -> Scope1/3

== system PV_MEV/EV System/PFC Control/Half Cycle Model Prediction ==
  u : Inport
  Constant1 : Constant  Value=0.01
  Data Type Conversion : DataTypeConversion  SaturateOnIntegerOverflow=off  RndMeth=Floor
  Data Type Conversion1 : DataTypeConversion  SaturateOnIntegerOverflow=off  RndMeth=Floor
  Data Type Conversion2 : DataTypeConversion  SaturateOnIntegerOverflow=off  RndMeth=Floor
  Demux : Demux  Outputs=7
  MATLAB Function : MATLAB Function  TreatAsAtomicUnit=on
  MATLAB Function3 : MATLAB Function  TreatAsAtomicUnit=on
  Mux1 : Mux  Inputs=3
  Mux6 : Mux
  ONNX Model Predict : pycoexlib/ONNX Model Predict  ModelFile=/home/changhong/prj/finn_cli_fork/scripts/HIL/HarmonicAI_Simulation/Model_Training2/harmonic_brevitas_run_half_opt/brevitas_harmonic_mlp.onnx  ExecutionProviders=CPUExecutionProvider  InputTable={ 'input', 'float32', '', '2' }  OutputTable={ 'output', '', '' }  SampleTime=1/2000  InputDatatypes=float32  InputNumDims=2  InputPermutations=[]  OutputPermutations=[]  PythonCoexecutionBlockType=ONNXModelBlock  VariableOutputMaxSizes=[]
  Sampling1 : ZeroOrderHold  SampleTime=1/2000
  Transpose : Math  Operator=transpose
  u_buff : Buffer  N=40  V=39  OutputFrames=off
  amplitude : Outport
  phase : Outport  Port=2
  wires:
  Transpose/1 -> MATLAB Function/1(x)
  u_buff/1 -> Transpose/1
  u/1 -> Sampling1/1
  Mux1/1 -> phase/1
  Mux6/1 -> amplitude/1
  Data Type Conversion2/1 -> Demux/1
  MATLAB Function3/1(y_post) -> Data Type Conversion2/1
  Demux/1 -> Mux6/1
  Demux/2 -> Mux6/2
  Demux/3 -> Mux6/3
  Demux/4 -> Mux6/4
  Demux/5 -> Mux1/1
  Demux/6 -> Mux1/2
  Demux/7 -> Mux1/3
  MATLAB Function/2(A) -> MATLAB Function3/2(A_latest)
  Constant1/1 -> MATLAB Function3/3(alpha)
  Data Type Conversion1/1 -> MATLAB Function3/1(y_rel)
  ONNX Model Predict/1 -> Data Type Conversion1/1
  Data Type Conversion/1 -> ONNX Model Predict/1
  MATLAB Function/1(x_norm) -> Data Type Conversion/1
  Sampling1/1 -> u_buff/1

== system PV_MEV/EV System/PFC Control/One  Cycle Model Prediction ==
  u : Inport
  Constant1 : Constant  Value=0.05
  Data Type Conversion : DataTypeConversion  SaturateOnIntegerOverflow=off  RndMeth=Floor
  Data Type Conversion1 : DataTypeConversion  SaturateOnIntegerOverflow=off  RndMeth=Floor
  Data Type Conversion2 : DataTypeConversion  SaturateOnIntegerOverflow=off  RndMeth=Floor
  Demux : Demux  Outputs=7
  MATLAB Function : MATLAB Function  TreatAsAtomicUnit=on
  MATLAB Function3 : MATLAB Function  TreatAsAtomicUnit=on
  Mux1 : Mux  Inputs=3
  Mux6 : Mux
  ONNX Model Predict : pycoexlib/ONNX Model Predict  ModelFile=/home/changhong/prj/finn_cli_fork/scripts/HIL/HarmonicAI_Simulation/Model_Training2/harmonic_brevitas_run_1cycle/brevitas_harmonic_mlp.onnx  ExecutionProviders=AzureExecutionProvider, CPUExecutionProvider  InputTable={ 'input', 'float32', '', '2' }  OutputTable={ 'output', '', '' }  SampleTime=1/4000  InputDatatypes=float32  InputNumDims=2  InputPermutations=[]  OutputPermutations=[]  PythonCoexecutionBlockType=ONNXModelBlock  VariableOutputMaxSizes=[]
  Sampling1 : ZeroOrderHold  SampleTime=1/(mm_fund_freq*mm_points_per_cycle)
  Transpose : Math  Operator=transpose
  u_buff : Buffer  N=mm_points_per_cycle  V=mm_sampling_overlap  OutputFrames=off
  amplitude : Outport
  phase : Outport  Port=2
  wires:
  Sampling1/1 -> u_buff/1
  MATLAB Function/1(x_norm) -> Data Type Conversion/1
  Data Type Conversion/1 -> ONNX Model Predict/1
  ONNX Model Predict/1 -> Data Type Conversion1/1
  Data Type Conversion1/1 -> MATLAB Function3/1(y_rel)
  Constant1/1 -> MATLAB Function3/3(alpha)
  MATLAB Function/2(A) -> MATLAB Function3/2(A_latest)
  Demux/7 -> Mux1/3
  Demux/6 -> Mux1/2
  Demux/5 -> Mux1/1
  Demux/4 -> Mux6/4
  Demux/3 -> Mux6/3
  Demux/2 -> Mux6/2
  Demux/1 -> Mux6/1
  MATLAB Function3/1(y_post) -> Data Type Conversion2/1
  Data Type Conversion2/1 -> Demux/1
  Mux6/1 -> amplitude/1
  Mux1/1 -> phase/1
  u/1 -> Sampling1/1
  u_buff/1 -> Transpose/1
  Transpose/1 -> MATLAB Function/1(x)

== system PV_MEV/EV System/PFC Control/PR2 ==
  Iref : Inport
  Iac : Inport  Port=2
  Gain : Gain  Gain=Kp
  Gain1 : Gain  Gain=Kr
  Second-Order Filter1 : spsSecondOrderFilterLib/Second-Order Filter  FilterType=Bandpass  Fo=Fr  Zeta=Zeta_I  Ts=Ts_Control  Initialize=off  Vac_Init="[0,  0,  60]"  Vdc_Init=0  PlotResponse=off  FreqRange=[0, 1000, 0.2]
  Sum1 : Sum  Inputs=|+-
  Sum2 : Sum  Inputs=|++
  D : Outport
  wires:
  Gain1/1 -> Second-Order Filter1/1
  Sum2/1 -> D/1
  Gain/1 -> Sum2/1
  Iac/1 -> Sum1/2
  Iref/1 -> Sum1/1
  Sum1/1 -> Gain1/1, Gain/1
  Second-Order Filter1/1 -> Sum2/2

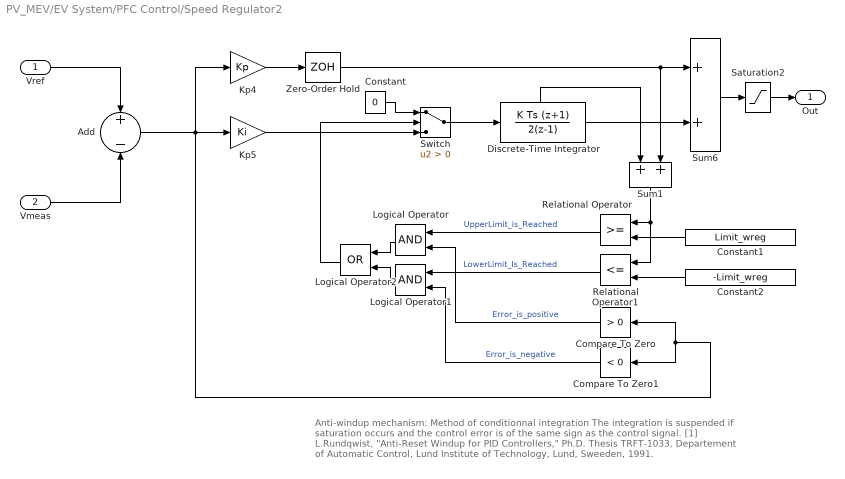
== system PV_MEV/EV System/PFC Control/Speed Regulator2 ==
  note: Anti-windup mechanism: Method of conditionnal integration
      |
      | The integration is suspended if saturation occurs and the
      | control error is of the same sign as the control signal.
      |
      | [1] L.Rundqwist, "Anti-Reset Windup for PID Controllers," Ph.D. Thesis TRFT-1033,
      | Departement of Automatic Control, Lund Institute of Technology, Lund, Sweeden, 1991.
  Vref : Inport  PortDimensions=1
  Vmeas : Inport  Port=2  PortDimensions=1
  Add : Sum  Inputs=+|-
  Compare To Zero : simulink/Logic and Bit Operations/Compare To Zero  relop=>  OutDataTypeStr=uint8  ZeroCross=off
  Compare To Zero1 : simulink/Logic and Bit Operations/Compare To Zero  relop=<  OutDataTypeStr=uint8  ZeroCross=off
  Constant : Constant  Value=0
  Constant1 : Constant  Value=Limit_wreg
  Constant2 : Constant  Value=-Limit_wreg
  Discrete-Time Integrator : DiscreteIntegrator  IntegratorMethod=Integration: Trapezoidal  InitialCondition=Init  SampleTime=Ts  LimitOutput=on  UpperSaturationLimit=Limit_wreg  LowerSaturationLimit=-Limit_wreg  ShowStatePort=on  ICPrevOutput=DiscIntNeverNeededParam  ICPrevScaledInput=DiscIntNeverNeededParam
  Kp4 : Gain  Gain=Kp  SaturateOnIntegerOverflow=on  SampleTime=Ts  OutDataTypeStr=Inherit: Same as input  ParamDataTypeStr=Inherit: Same as input
  Kp5 : Gain  Gain=Ki  SaturateOnIntegerOverflow=on  SampleTime=Ts  OutDataTypeStr=Inherit: Same as input  ParamDataTypeStr=Inherit: Same as input
  Logical Operator : Logic  AllPortsSameDT=off  OutDataTypeStr=boolean
  Logical Operator1 : Logic  AllPortsSameDT=off  OutDataTypeStr=boolean
  Logical Operator2 : Logic  Operator=OR  AllPortsSameDT=off  OutDataTypeStr=boolean
  Relational Operator : RelationalOperator  OutDataTypeStr=boolean  InputSameDT=off
  Relational Operator1 : RelationalOperator  Operator=<=  OutDataTypeStr=boolean  InputSameDT=off
  Saturation2 : Saturate  UpperLimit=Limit_wreg  LowerLimit=-Limit_wreg  SampleTime=Ts
  Sum1 : Sum  InputSameDT=on  SaturateOnIntegerOverflow=on  SampleTime=Ts  OutDataTypeStr=Inherit: Same as first input
  Sum6 : Sum  InputSameDT=on  SaturateOnIntegerOverflow=on  SampleTime=Ts  OutDataTypeStr=Inherit: Same as first input
  Switch : Switch  Criteria=u2 > Threshold  SaturateOnIntegerOverflow=off  InputSameDT=off
  Zero-Order Hold : ZeroOrderHold  SampleTime=Ts
  Out : Outport  SampleTime=Ts  InitialOutput=0  VectorParamsAs1DForOutWhenUnconnected=off
  wires:
  Kp5/1 -> Switch/3
  Switch/1 -> Discrete-Time Integrator/1
  Saturation2/1 -> Out/1
  Discrete-Time Integrator/1 -> Sum6/2
  Kp4/1 -> Zero-Order Hold/1
  Sum6/1 -> Saturation2/1
  Add/1 -> Compare To Zero/1, Compare To Zero1/1, Kp5/1, Kp4/1
  Compare To Zero1/1 -> Logical Operator1/2  "Error_is_negative"
  Logical Operator1/1 -> Logical Operator2/2
  Logical Operator/1 -> Logical Operator2/1
  Compare To Zero/1 -> Logical Operator/2  "Error_is_positive"
  Constant2/1 -> Relational Operator1/2
  Constant1/1 -> Relational Operator/2
  Relational Operator1/1 -> Logical Operator1/1  "LowerLimit_Is_Reached"
  Relational Operator/1 -> Logical Operator/1  "UpperLimit_is_Reached"
  Logical Operator2/1 -> Switch/2
  Sum1/1 -> Relational Operator/1, Relational Operator1/1
  Discrete-Time Integrator/State -> Sum1/1
  Zero-Order Hold/1 -> Sum6/1, Sum1/2
  Constant/1 -> Switch/1
  Vref/1 -> Add/1
  Vmeas/1 -> Add/2

== system PV_MEV/EV System/PFC Control/fft estimation 1 cycle2 ==
  u : Inport
  Buffer 1cycle : Buffer  N=mm_points_per_cycle  V=mm_sampling_overlap  OutputFrames=off
  Constant4 : Constant  Value=mm_fund_freq
  Constant5 : Constant  Value=mm_points_per_cycle * mm_fund_freq
  FFT_estimation_1 : MATLAB Function  TreatAsAtomicUnit=on
  Sampling : ZeroOrderHold  SampleTime=1/(mm_fund_freq*mm_points_per_cycle)
  amp : Outport
  phase : Outport  Port=2
  wires:
  Sampling/1 -> Buffer 1cycle/1
  Buffer 1cycle/1 -> FFT_estimation_1/1(u)
  Constant5/1 -> FFT_estimation_1/2(fs)
  Constant4/1 -> FFT_estimation_1/3(f0)
  u/1 -> Sampling/1
  FFT_estimation_1/1(amp) -> amp/1
  FFT_estimation_1/2(phase) -> phase/1

== system PV_MEV/EV System/PFC Control/fft estimation 10 cycle2 ==
  u : Inport
  Buffer 10cycle : Buffer  N=mm_10cycle_points  V=mm_10cycle_overlap  OutputFrames=off
  Constant4 : Constant  Value=mm_fund_freq
  Constant5 : Constant  Value=mm_points_per_cycle * mm_fund_freq
  FFT_estimation : MATLAB Function  TreatAsAtomicUnit=on
  Sampling : ZeroOrderHold  SampleTime=1/(mm_fund_freq*mm_points_per_cycle)
  amp : Outport
  phase : Outport  Port=2
  wires:
  FFT_estimation/2(phase) -> phase/1
  FFT_estimation/1(amp) -> amp/1
  u/1 -> Sampling/1
  Constant4/1 -> FFT_estimation/3(f0)
  Constant5/1 -> FFT_estimation/2(fs)
  Buffer 10cycle/1 -> FFT_estimation/1(u)
  Sampling/1 -> Buffer 10cycle/1

== system PV_MEV/EV System1/PFC Control/Half Cycle Model Prediction ==
  u : Inport
  Constant1 : Constant  Value=0.01
  Data Type Conversion : DataTypeConversion  SaturateOnIntegerOverflow=off  RndMeth=Floor
  Data Type Conversion1 : DataTypeConversion  SaturateOnIntegerOverflow=off  RndMeth=Floor
  Data Type Conversion2 : DataTypeConversion  SaturateOnIntegerOverflow=off  RndMeth=Floor
  Demux : Demux  Outputs=7
  MATLAB Function : MATLAB Function  TreatAsAtomicUnit=on
  MATLAB Function3 : MATLAB Function  TreatAsAtomicUnit=on
  Mux1 : Mux  Inputs=3
  Mux6 : Mux
  ONNX Model Predict : pycoexlib/ONNX Model Predict  ModelFile=/home/changhong/prj/finn_cli_fork/scripts/HIL/HarmonicAI_Simulation/Model_Training2/harmonic_brevitas_run_half_opt/brevitas_harmonic_mlp.onnx  ExecutionProviders=CPUExecutionProvider  InputTable={ 'input', 'float32', '', '2' }  OutputTable={ 'output', '', '' }  SampleTime=1/2000  InputDatatypes=float32  InputNumDims=2  InputPermutations=[]  OutputPermutations=[]  PythonCoexecutionBlockType=ONNXModelBlock  VariableOutputMaxSizes=[]
  Sampling1 : ZeroOrderHold  SampleTime=1/2000
  Transpose : Math  Operator=transpose
  u_buff : Buffer  N=40  V=39  OutputFrames=off
  amplitude : Outport
  phase : Outport  Port=2
  wires:
  Sampling1/1 -> u_buff/1
  MATLAB Function/1(x_norm) -> Data Type Conversion/1
  Data Type Conversion/1 -> ONNX Model Predict/1
  ONNX Model Predict/1 -> Data Type Conversion1/1
  Data Type Conversion1/1 -> MATLAB Function3/1(y_rel)
  Constant1/1 -> MATLAB Function3/3(alpha)
  MATLAB Function/2(A) -> MATLAB Function3/2(A_latest)
  Demux/7 -> Mux1/3
  Demux/6 -> Mux1/2
  Demux/5 -> Mux1/1
  Demux/4 -> Mux6/4
  Demux/3 -> Mux6/3
  Demux/2 -> Mux6/2
  Demux/1 -> Mux6/1
  MATLAB Function3/1(y_post) -> Data Type Conversion2/1
  Data Type Conversion2/1 -> Demux/1
  Mux6/1 -> amplitude/1
  Mux1/1 -> phase/1
  u/1 -> Sampling1/1
  u_buff/1 -> Transpose/1
  Transpose/1 -> MATLAB Function/1(x)

== system PV_MEV/EV System1/PFC Control/One  Cycle Model Prediction ==
  u : Inport
  Constant1 : Constant  Value=0.05
  Data Type Conversion : DataTypeConversion  SaturateOnIntegerOverflow=off  RndMeth=Floor
  Data Type Conversion1 : DataTypeConversion  SaturateOnIntegerOverflow=off  RndMeth=Floor
  Data Type Conversion2 : DataTypeConversion  SaturateOnIntegerOverflow=off  RndMeth=Floor
  Demux : Demux  Outputs=7
  MATLAB Function : MATLAB Function  TreatAsAtomicUnit=on
  MATLAB Function3 : MATLAB Function  TreatAsAtomicUnit=on
  Mux1 : Mux  Inputs=3
  Mux6 : Mux
  ONNX Model Predict : pycoexlib/ONNX Model Predict  ModelFile=/home/changhong/prj/finn_cli_fork/scripts/HIL/HarmonicAI_Simulation/Model_Training2/harmonic_brevitas_run_1cycle/brevitas_harmonic_mlp.onnx  ExecutionProviders=AzureExecutionProvider, CPUExecutionProvider  InputTable={ 'input', 'float32', '', '2' }  OutputTable={ 'output', '', '' }  SampleTime=1/4000  InputDatatypes=float32  InputNumDims=2  InputPermutations=[]  OutputPermutations=[]  PythonCoexecutionBlockType=ONNXModelBlock  VariableOutputMaxSizes=[]
  Sampling1 : ZeroOrderHold  SampleTime=1/(mm_fund_freq*mm_points_per_cycle)
  Transpose : Math  Operator=transpose
  u_buff : Buffer  N=mm_points_per_cycle  V=mm_sampling_overlap  OutputFrames=off
  amplitude : Outport
  phase : Outport  Port=2
  wires:
  Transpose/1 -> MATLAB Function/1(x)
  u_buff/1 -> Transpose/1
  u/1 -> Sampling1/1
  Mux1/1 -> phase/1
  Mux6/1 -> amplitude/1
  Data Type Conversion2/1 -> Demux/1
  MATLAB Function3/1(y_post) -> Data Type Conversion2/1
  Demux/1 -> Mux6/1
  Demux/2 -> Mux6/2
  Demux/3 -> Mux6/3
  Demux/4 -> Mux6/4
  Demux/5 -> Mux1/1
  Demux/6 -> Mux1/2
  Demux/7 -> Mux1/3
  MATLAB Function/2(A) -> MATLAB Function3/2(A_latest)
  Constant1/1 -> MATLAB Function3/3(alpha)
  Data Type Conversion1/1 -> MATLAB Function3/1(y_rel)
  ONNX Model Predict/1 -> Data Type Conversion1/1
  Data Type Conversion/1 -> ONNX Model Predict/1
  MATLAB Function/1(x_norm) -> Data Type Conversion/1
  Sampling1/1 -> u_buff/1

== system PV_MEV/EV System1/PFC Control/PR2 ==
  Iref : Inport
  Iac : Inport  Port=2
  Gain : Gain  Gain=Kp
  Gain1 : Gain  Gain=Kr
  Second-Order Filter1 : spsSecondOrderFilterLib/Second-Order Filter  FilterType=Bandpass  Fo=Fr  Zeta=Zeta_I  Ts=Ts_Control  Initialize=off  Vac_Init="[0,  0,  60]"  Vdc_Init=0  PlotResponse=off  FreqRange=[0, 1000, 0.2]
  Sum1 : Sum  Inputs=|+-
  Sum2 : Sum  Inputs=|++
  D : Outport
  wires:
  Second-Order Filter1/1 -> Sum2/2
  Sum1/1 -> Gain/1, Gain1/1
  Iref/1 -> Sum1/1
  Iac/1 -> Sum1/2
  Gain/1 -> Sum2/1
  Sum2/1 -> D/1
  Gain1/1 -> Second-Order Filter1/1
